simulink model "Assignment_1_b"  (R2021a)
settings: Solver=VariableStepAuto  StartTime=0.0  StopTime=10.0  RelTol=1e-3
undefined symbols (not defined in the file): c1, c2, k1, k2, m1, m2
settings Model: Creator=hp  LastModifiedBy=hp

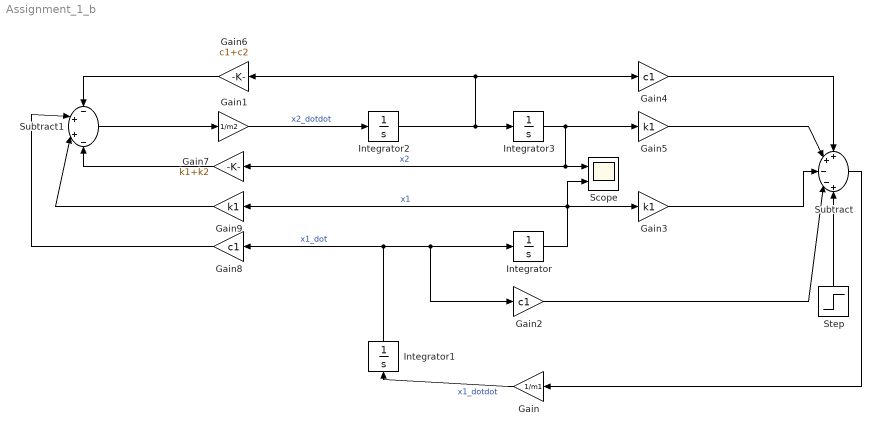
== system Assignment_1_b ==
  Gain : Gain  Gain=1/m1
  Gain1 : Gain  Gain=1/m2
  Gain2 : Gain  Gain=c1
  Gain3 : Gain  Gain=k1
  Gain4 : Gain  Gain=c1
  Gain5 : Gain  Gain=k1
  Gain6 : Gain  Gain=c1+c2
  Gain7 : Gain  Gain=k1+k2
  Gain8 : Gain  Gain=c1
  Gain9 : Gain  Gain=k1
  Integrator{,1..3} (4 alike) : Integrator
  Scope : Scope  NumInputPorts=2
  Step : Step  After=5  SampleTime=0
  Subtract : Sum  Inputs=++--+
  Subtract1 : Sum  Inputs=-++-
  wires:
  Gain/1 -> Integrator1/1  "x1_dotdot"
  Integrator1/1 -> Gain8/1, Gain2/1, Integrator/1  "x1_dot"
  Integrator/1 -> Scope/2, Gain3/1, Gain9/1  "x1"
  Gain1/1 -> Integrator2/1  "x2_dotdot"
  Integrator2/1 -> Gain4/1, Gain6/1, Integrator3/1
  Integrator3/1 -> Scope/1, Gain7/1, Gain5/1  "x2"
  Subtract/1 -> Gain/1
  Gain2/1 -> Subtract/4
  Gain3/1 -> Subtract/3
  Gain4/1 -> Subtract/1
  Gain5/1 -> Subtract/2
  Gain6/1 -> Subtract1/1
  Gain7/1 -> Subtract1/4
  Gain8/1 -> Subtract1/2
  Gain9/1 -> Subtract1/3
  Subtract1/1 -> Gain1/1
  Step/1 -> Subtract/5
